simulink model "ERES_PIMC_Controller_Simulation"  (R2018a)
settings: Solver=VariableStepAuto  StartTime=0.0  StopTime=120  RelTol=1e-3
undefined symbols (not defined in the file): a_lateral_max, atableall, feedback_filter_limit_max, feedback_filter_limit_min, fl_x, fl_y, fr_x, fr_y, friction_table, imc_acc_error_coeffi, integrator_saturation_level, Ki, num, proportion, proportion_loop_limit, speed_controller_input_limit, station_error_limit, station_integrator_saturation_level, station_Ki, station_Kp, steer_angle_limited, steer_ratio, T7_with_trailer_atable, T7_with_trailer_atableall, T7_with_trailer_engine_speed_table, T7_with_trailer_engine_throttle_table, T7_with_trailer_engine_torqe_tableall, T7_with_trailer_utable, T7_with_trailer_utableall, T7_with_trailer_vtable, t_delay, throttle_table, utable, v_table, Vr, vtable, w1, w2, wheel_base, x0, y0
libraries: simulink x2, Solver_SF x1
(part 2 of 2)

== matlab function ERES_PIMC_Controller_Simulation/mass_estimateV2.0/feedforward filter/feedforward filter ==
  data: a_d input; belta input; a_df output; a_df_1 input
function a_df = fcn(a_d,belta,a_df_1)

a_df = belta * a_df_1 + ( 1 - belta) * a_d;

== matlab function ERES_PIMC_Controller_Simulation/mass_estimateV3.0/M_Trans_filter1/feedforward filter1/feedforward filter ==
  data: a_d input; belta input; a_df output; a_df_1 input
function a_df = fcn(a_d,belta,a_df_1)

a_df = belta * a_df_1 + ( 1 - belta) * a_d;

== matlab function ERES_PIMC_Controller_Simulation/mass_estimateV2.0/mass estimate ==
  data: friction input; mass output; F_air input; Iw_Dr_L1 input; Iw_Dr_L2 input; Iw_Dr_L3 input; Iw_Dr_L4 input; Iw_Dr_L5 input; brake input; M_Trans input; pitch input; vx input; noise input; w input; ac input; mass_k_1 input; p_k_1 input; K_k_1 input; P output; K output; phi output; Fg output; tmp output
function [mass,P,K,phi,Fg,tmp] = fcn(friction,F_air,Iw_Dr_L1,Iw_Dr_L2,Iw_Dr_L3,Iw_Dr_L4,Iw_Dr_L5,brake,...
                                                        M_Trans,pitch,vx,noise,w,ac,mass_k_1,p_k_1,K_k_1)
% Fc = 0;theta = 0;Ft = 0;
na = 1;nb = 1;d = 3; %structure parameters
ig = 0.92;
i0 = 4.4;
yita = 0.9;
f0 = 0.0006;
f1 = 0.000028273;
g = 9.8;%unit:m/s^2
r = 0.535;

keci = 1 + (Iw_Dr_L1 + Iw_Dr_L2 + Iw_Dr_L3 + Iw_Dr_L4 + Iw_Dr_L5 )/ r^2;
tmp = g * (f0 + f1 * vx * 3.6);

Ft = M_Trans * ig * i0 * yita / r;
Fg = Ft + F_air + brake;
% if ac >= 0
%     phi = g * pitch + g * (f0 + f1 * vx) + ac+ noise;
% else
%     phi = g * pitch + g * (f0 + f1 * vx) - ac+ noise;
% end
phi = g * pitch +  g * friction+ ac+ noise*1;
% Ft = M_Trans * ig * i0 * yita / r;
% Fg = Ft + F_air;
% mass = 0;% initial value of the object to be estimated
% persistent mass_last;
% mass_last = 0;
% P = 10^6 * eye(na - 1 + nb - 1 + 1);
% Fg = phi * m + xi; % y(k) = phi(k-1)' * theta + xi 标准的最小二乘形式
% mass_k_1  = 10000; 

% RLS algorithm
K = p_k_1 * phi / (w + phi' * p_k_1 * phi);
% mass = mass_last + K * (Fg - phi' * mass_last);
mass = mass_k_1 + K * (Fg - phi' * mass_k_1);
% mass = mass_k_1 + K_k_1 * (Fg - phi' * mass_k_1);
P =1 / w * (eye(na - 1 + nb - 1 + 1) - K * phi') * p_k_1;%K_k_1
% P =1 / w * (eye(na - 1 + nb - 1 + 1) - K_k_1 * phi') * p_k_1;%K_k_1
% P =1 / w * (p_k_1 -  p_k_1 * phi  / ( w + phi' *  p_k_1 * phi) * phi' *p_k_1) ;
% if mass <=0
%     mass = 0;
% end

% mass_last = mass;

== matlab function ERES_PIMC_Controller_Simulation/mass_estimateV1.0/feedforward filter1/feedforward filter ==
  data: a_d input; belta input; a_df output; a_df_1 input
function a_df = fcn(a_d,belta,a_df_1)

a_df = belta * a_df_1 + ( 1 - belta) * a_d;

== matlab function ERES_PIMC_Controller_Simulation/Longitude P-IMC controller/feedback filter1/feedback filter ==
  data: a_d input; belta input; a_df output; a_df_1 input
function a_df = fcn(a_d,belta,a_df_1)

a_df = belta * a_df_1 + ( 1 - belta) * a_d;

== matlab function ERES_PIMC_Controller_Simulation/mass_estimateV3.0/feedforward filter/feedforward filter ==
  data: a_d input; belta input; a_df output; a_df_1 input
function a_df = fcn(a_d,belta,a_df_1)

a_df = belta * a_df_1 + ( 1 - belta) * a_d;

== matlab function ERES_PIMC_Controller_Simulation/mass_estimateV3.0/mass estimate ==
  data: friction input; mass output; F_air input; Iw_Dr_L1 input; Iw_Dr_L2 input; Iw_Dr_L3 input; Iw_Dr_L4 input; Iw_Dr_L5 input; brake input; M_Trans input; pitch input; vx input; noise input; w input; ac input; mass_k_1 input; p_k_1 input; K_k_1 input; P output; K output; phi output; Fg output; tmp output
function [mass,P,K,phi,Fg,tmp] = fcn(friction,F_air,Iw_Dr_L1,Iw_Dr_L2,Iw_Dr_L3,Iw_Dr_L4,Iw_Dr_L5,brake,...
                                                        M_Trans,pitch,vx,noise,w,ac,mass_k_1,p_k_1,K_k_1)
% Fc = 0;theta = 0;Ft = 0;
na = 1;nb = 1;d = 3; %structure parameters
ig = 0.92;
i0 = 4.4;
yita = 0.9;
f0 = 0.0006;
f1 = 0.000028273;
g = 9.8;%unit:m/s^2
r = 0.535;
F_R = 0;% F_R = F_air + F_res;这里把F_R看成是阻力的集合
theta = [];
phi = [];


keci = 1 + (Iw_Dr_L1 + Iw_Dr_L2 + Iw_Dr_L3 + Iw_Dr_L4 + Iw_Dr_L5 )/ r^2;
tmp = g * (f0 + f1 * vx * 3.6);

Ft = M_Trans * ig * i0 * yita / r;
% Fg = Ft + F_air + brake;
Fg = Ft ;



% phi = g * pitch +  g * friction+ ac+ noise*1;
a_sensor = g * pitch + ac+ noise*1;
phi = [a_sensor 1];
theta = [mass F_R];
% Ft = M_Trans * ig * i0 * yita / r;
% Fg = Ft + F_air;
% mass = 0;% initial value of the object to be estimated
% persistent mass_last;
% mass_last = 0;
% P = 10^6 * eye(na - 1 + nb - 1 + 1);
% Fg = phi * m + xi; % y(k) = phi(k-1)' * theta + xi 标准的最小二乘形式
% mass_k_1  = 10000; 

% RLS algorithm
% K = p_k_1 * phi / (w + phi' * p_k_1 * phi);
% 
% mass = mass_k_1 + K * (Fg - phi' * mass_k_1);
% 
% P =1 / w * (eye(na - 1 + nb - 1 + 1) - K * phi') * p_k_1;%K_k_1
K = p_k_1 * phi / (w + phi' * p_k_1 * phi);

mass = mass_k_1 + K * (Fg - phi' * mass_k_1);

P =1 / w * (eye(na - 1 + nb - 1 + 1) - K * phi') * p_k_1;%K_k_1





% mass_last = mass;

== matlab function ERES_PIMC_Controller_Simulation/mass_estimateV2.0/M_Trans_filter1/feedforward filter1/feedforward filter ==
  data: a_d input; belta input; a_df output; a_df_1 input
function a_df = fcn(a_d,belta,a_df_1)

a_df = belta * a_df_1 + ( 1 - belta) * a_d;
